simulink library "commfilt2"  (Simulink 6.0)
settings: Solver=ode45  SolverMode=SingleTasking  StartTime=0.0  StopTime=10.0  RelTol=1e-3
undefined symbols (not defined in the file or in its folder): hFilt, rectPul
libraries: dspsigattribs x6, dsparch4 x3, dspsigops x3, dspmlti3 x1
settings Model: Creator=arodrigu  LastModifiedBy=cvora  ExtModeAutoUpdateStatusClock=off  ProdHWDeviceType=Specified
settings DataIOCC: SignalLoggingName=logsOut
settings OptimizationCC: BooleanDataType=off
settings DebuggingCC: CheckExecutionContextPreStartOutputMsg=on  CheckExecutionContextRuntimeOutputMsg=on  SolverPrmCheckMsg=none
settings HardwareCC: ProdHWDeviceType=Specified  TargetUnknown=on
settings ModelReferenceCC: UpdateModelReferenceTargets=IfOutOfDate
settings SFSimCC: SFSimApplyToAllLibs=on  SFSimBuildMode=Incremental

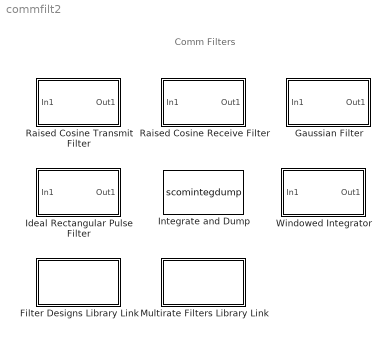
== system commfilt2 ==
  note: Comm Filters
  Filter Designs Library Link : Subsystem  PropExecContextAcrossSSBoundary=on  mask(Link to Filter Designs Library){myFiltDesignsParam=0}
      mask prompts: myFiltDesignsParam "option:"
      settings: OpenFcn=commblkmorefilt('dsparch');
      mask Display: disp('Filter\n Designs Link');
  Gaussian Filter : Subsystem  PropExecContextAcrossSSBoundary=on  mask(Gaussian Filter){N=8, BT=0.3, D=2, sampMode=Frame-based, normMode=Sum of coefficients, filterGain=1, checkCoeff=Off, variableName=gaussFilt, launchFVT=Off}
      mask prompts: N "Input samples per symbol (N):"; BT "BT product:"; D "Group delay (number of symbols):"; sampMode "Input sampling mode:"; normMode "Filter coefficient normalization:"; filterGain "Linear amplitude filter gain:"; checkCoeff "Export filter coefficients to workspace"; variableName "Coefficient variable name:"; launchFVT "Launch Filter Visualization Tool (FVTool)"
      mask help:
      | Filter the input signal using a Gaussian FIR filter.
      |
      | The group delay is specified as the number of symbol periods between the start of the filter response and its peak. This delay also determines the length of the filter impulse response, which is 2 * N * Group delay + 1.
      mask init:
      | [hFilt,icon,msg] = commblkgaussfilt(gcb,'init');
      | if(~isempty(msg))
      | 	error(msg);
      | end
      | 
      | %-- Open FVtool
      | if strcmp(get_param(bdroot(gcb),'simulationstatus'),'stopped')
      | lnkfvtool2mask(gcb);
      | end
      settings: CopyFcn=commblkgaussfilt(gcb,'cbCopyFcn');
      mask Help: helpview(commbhelp);
      mask StyleString: edit,edit,edit,popup(Frame-based|Sample-based),popup(Sum of coefficients|Filter energy|Peak amplitude),edit,checkbox,edit,checkbox
      mask CallbackString: |||commblkgaussfilt(gcb,'cbSampMode');|||commblkgaussfilt(gcb,'cbCheckCoeff');||
      mask Display: plot(0,0,1,1,icon.xx,icon.plot); text(icon.x,icon.y,icon.str,'horiz','center');
  Ideal Rectangular Pulse Filter : Subsystem  PropExecContextAcrossSSBoundary=on  mask(Ideal Rectangular Pulse Filter){pulseLen=8, pulseDelay=0, sampMode=Frame-based, normCheck=on, normMode=Sum of samples, filterGain=1}
      mask prompts: pulseLen "Pulse length (number of samples):"; pulseDelay "Pulse delay (number of samples):"; sampMode "Input sampling mode:"; normCheck "Normalize output signal"; normMode "Normalization method:"; filterGain "Linear amplitude gain:"
      mask help:
      | Upsample the input signal using ideal rectangular pulses.
      |
      | This block replicates each input sample N times, where N is the pulse length. This block can also normalize the output signal and apply a linear amplitude gain.
      mask init:
      | [rectPul,msg] = commblkrectpulse(gcb,'init');
      | if(~isempty(msg))
      | 	error(msg);
      | end
      settings: CopyFcn=commblkrectpulse(gcb,'cbCopyFcn');
      mask Help: helpview(commbhelp);
      mask StyleString: edit,edit,popup(Frame-based|Sample-based),checkbox,popup(Sum of samples|Energy per pulse),edit
      mask CallbackString: ||commblkrectpulse(gcb,'cbSampMode');|commblkrectpulse(gcb,'cbNormCheck');||
      mask Display:
      | plot(0,0,100,100,[95 5 10 10 10 reshape(([85*[0:1/15:1-1/15]+10; 85*[1/15:1/15:1]+10]),1,30)],[75 75 75 70 95 90 90 90 90 90 90 90 90 80 80 80 80 80 80 80 80 80 80 90 90 90 90 90 90 90 90 80 80 80 80]*1.1-10);
      | text(50,35,'Rectangular\nPulse Filter','horiz','center');
  Integrate and Dump : S-Function  FunctionName=scomintegdump  Parameters=obssamples, offsetsamples, nodump  mask(Integrate and dump){obssamples=8, offsetsamples=0, nodump=off}
      mask prompts: obssamples "Integration period (number of samples):"; offsetsamples "Offset (number of samples):"; nodump "Output intermediate values"
      mask help:
      | Integrate over number of samples in integration period and reset at the end of integration.
      |
      | Frame based K x L input is treated as L channels each of frame size K.
      | The samples are integrated along every column.
      |
      | Offset samples are ignored during the first integration period.
      mask Help: helpview(commbhelp);
      mask Display: disp('Integrate\nand Dump')
  Multirate Filters Library Link : Subsystem  PropExecContextAcrossSSBoundary=on  mask(Link to Multirate Filters Library){myMultirateFiltersParam=0}
      mask prompts: myMultirateFiltersParam "option:"
      settings: OpenFcn=commblkmorefilt('dspmlti');
      mask Display: disp('Multirate\nFilters Link');
  Raised Cosine Receive Filter : Subsystem  PropExecContextAcrossSSBoundary=on  mask(Raised Cosine Receive Filter){filtType=Square root, N=8, D=4, R=0.2, sampMode=Frame-based, rateMode=Downsampling, downFactor=8, downOffset=0, checkGain=Normalized, filterGain=1, checkCoeff=off, variableName=rcRxFilt, launchFVT=off}
      mask prompts: filtType "Filter type:"; N "Input samples per symbol (N):"; D "Group delay (number of symbols):"; R "Rolloff factor (0 to 1):"; sampMode "Input sampling mode:"; rateMode "Output mode:"; downFactor "Downsampling factor (L):"; downOffset "Sample offset (0 to L-1):"; checkGain "Filter gain:"; filterGain "Linear amplitude filter gain:"; checkCoeff "Export filter coefficients to workspace"; variableName "Coefficient variable name:"; launchFVT "Launch Filter Visualization Tool (FVTool)"
      mask help:
      | Filter the input signal, and downsample if selected, using a normal or square root raised cosine FIR filter.
      |
      | The group delay is specified as the number of symbol periods between the start of the filter response and its peak. This delay also determines the length of the filter impulse response, which is 2 * N * Group delay + 1.
      |
      | In normalized mode, the coefficients of the normal raised cosine filter are normalized so that the peak coefficient is equal to one. The filter coefficients of the square root raised cosine filter are normalized so that the impulse response of the filter convolved with itself is approximately the impulse response of the normal filter.
      mask init:
      | [hFilt,icon,msg] = commblkrcfilt(gcb,'init','RX');
      | if(~isempty(msg))
      | 	error(msg);
      | end
      | 
      | %-- Open FVtool
      | if strcmp(get_param(bdroot(gcb),'simulationstatus'),'stopped')
      | lnkfvtool2mask(gcb);
      | end
      settings: CopyFcn=commblkrcfilt(gcb,'cbCopyFcn');
      mask Help: helpview(commbhelp);
      mask StyleString: popup(Normal|Square root),edit,edit,edit,popup(Frame-based|Sample-based),popup(Downsampling|None),edit,edit,popup(Normalized|User-specified),edit,checkbox,edit,checkbox
      mask CallbackString: ||||commblkrcfilt(gcb,'cbSampMode','RX');|commblkrcfilt(gcb,'cbRateMode');|||commblkrcfilt(gcb,'cbCheckGain');||commblkrcfilt(gcb,'cbCheckCoeff');||
      mask Display: plot(0,0,1,1,icon.xx,icon.plot); text(icon.x,icon.y,icon.str,'horiz','center');
  Raised Cosine Transmit Filter : Subsystem  PropExecContextAcrossSSBoundary=on  mask(Raised Cosine Transmit Filter){filtType=Square root, D=4, R=0.2, sampMode=Frame-based, N=8, checkGain=Normalized, filterGain=1, checkCoeff=off, variableName=rcTxFilt, launchFVT=off}
      mask prompts: filtType "Filter type:"; D "Group delay (number of symbols):"; R "Rolloff factor (0 to 1):"; sampMode "Input sampling mode:"; N "Upsampling factor (N):"; checkGain "Filter gain:"; filterGain "Linear amplitude filter gain:"; checkCoeff "Export filter coefficients to workspace"; variableName "Coefficient variable name:"; launchFVT "Launch Filter Visualization Tool (FVTool)"
      mask help:
      | Upsample and filter the input signal using a normal or square root raised cosine FIR filter.
      |
      | The group delay is specified as the number of symbol periods between the start of the filter response and its peak. This delay also determines the length of the filter impulse response, which is 2 * N * Group delay + 1.
      |
      | In normalized mode, the coefficients of the normal raised cosine filter are normalized so that the peak coefficient is equal to one. The filter coefficients of the square root raised cosine filter are normalized so that the impulse response of the filter convolved with itself is approximately the impulse response of the normal filter.
      mask init:
      | [hFilt,icon,msg] = commblkrcfilt(gcb,'init','TX');
      | if(~isempty(msg))
      | 	error(msg);
      | end
      | 
      | %-- Open FVtool
      | if strcmp(get_param(bdroot(gcb),'simulationstatus'),'stopped')
      | lnkfvtool2mask(gcb);
      | end
      settings: CopyFcn=commblkrcfilt(gcb,'cbCopyFcn');
      mask Help: helpview(commbhelp);
      mask StyleString: popup(Normal|Square root),edit,edit,popup(Frame-based|Sample-based),edit,popup(Normalized|User-specified),edit,checkbox,edit,checkbox
      mask CallbackString: |||commblkrcfilt(gcb,'cbSampMode','TX');||commblkrcfilt(gcb,'cbCheckGain');||commblkrcfilt(gcb,'cbCheckCoeff');||
      mask Display: plot(0,0,1,1,icon.xx,icon.plot); text(icon.x,icon.y,icon.str,'horiz','center');
  Windowed Integrator : Subsystem  PropExecContextAcrossSSBoundary=on  mask(Windowed Integrator){integperiod=8}
      mask prompts: integperiod "Integration period (number of samples):"
      mask help: Integrate a discrete input signal over the sliding window of size equal to the integration period.
      mask init:
      | msg = commblkwininteg(gcb);
      | if(~isempty(msg))
      | 	error(msg);
      | end
      settings: ErrorFcn=commblkwinintegchk
      mask Help: helpview(commbhelp);
      mask Display: disp('Windowed\nIntegrator');

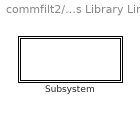
== system commfilt2/Filter Designs Library Link ==
  Subsystem : Subsystem  PropExecContextAcrossSSBoundary=on
      mask Display: disp(' ')

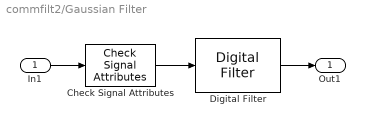
== system commfilt2/Gaussian Filter ==
  In1 : Inport  LatchInput=off
  Check Signal Attributes : dspsigattribs/Check Signal Attributes  SigAttribCheckMethod=Does not match attributes exactly  Complexity=Ignore  Frame=Frame-based  DimsCheckMethod=Is...  Dimensions=Column vector (2-D) or scalar  DatatypeCheckMethod=Ignore  DatatypeGeneral=Boolean  DtypeFloatSpecific=Any floating-point  DtypeFixedSpecific=Any fixed-point  DtypeIntSpecific=Any integer  SampleMode=Ignore
  Digital Filter : dsparch4/Digital Filter  TypePopup=FIR (all zeros)  IIRFiltStruct=Direct form II transposed  AllPoleFiltStruct=Direct form  FIRFiltStruct=Direct form  CoeffSource=Specify via dialog  NumCoeffs=hFilt.coeff  DenCoeffs=[1]  BiQuadCoeffs=[1 0.3 0.4 1 0.1 0.2]  LatticeCoeffs=[0.2 0.4]  denIgnore=on  FiltPerSampPopup=One filter per frame  IC=0  ICnum=0  ICden=0  roundingMode=Floor  overflowMode=off
  Out1 : Outport
  wires:
  Digital Filter/1 -> Out1/1
  Check Signal Attributes/1 -> Digital Filter/1
  In1/1 -> Check Signal Attributes/1

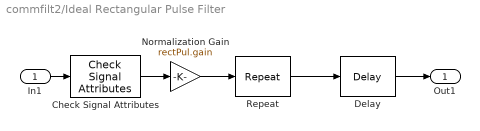
== system commfilt2/Ideal Rectangular Pulse Filter ==
  In1 : Inport  LatchInput=off
  Check Signal Attributes : dspsigattribs/Check Signal Attributes  SigAttribCheckMethod=Does not match attributes exactly  Complexity=Ignore  Frame=Frame-based  DimsCheckMethod=Is...  Dimensions=Column vector (2-D) or scalar  DatatypeCheckMethod=Ignore  DatatypeGeneral=Boolean  DtypeFloatSpecific=Any floating-point  DtypeFixedSpecific=Any fixed-point  DtypeIntSpecific=Any integer  SampleMode=Ignore
  Delay : dspsigops/Delay  dly_unit=Samples  delay=rectPul.pulseDelay  ic_detail=off  dif_ic_for_ch=off  dif_ic_for_dly=off  ic=0  reset_popup=None
  Normalization Gain : Gain  Gain=rectPul.gain  SaturateOnIntegerOverflow=on
  Repeat : dspsigops/Repeat  N=rectPul.pulseLen  ic=0  mode=Maintain input frame rate
  Out1 : Outport
  wires:
  Delay/1 -> Out1/1
  Normalization Gain/1 -> Repeat/1
  In1/1 -> Check Signal Attributes/1
  Repeat/1 -> Delay/1
  Check Signal Attributes/1 -> Normalization Gain/1

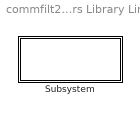
== system commfilt2/Multirate Filters Library Link ==
  Subsystem : Subsystem  PropExecContextAcrossSSBoundary=on
      mask Display: disp(' ')

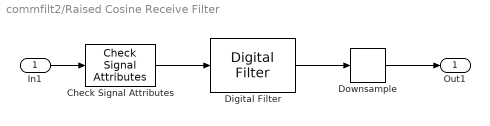
== system commfilt2/Raised Cosine Receive Filter ==
  In1 : Inport  LatchInput=off
  Check Signal Attributes : dspsigattribs/Check Signal Attributes  SigAttribCheckMethod=Does not match attributes exactly  Complexity=Ignore  Frame=Frame-based  DimsCheckMethod=Is...  Dimensions=Column vector (2-D) or scalar  DatatypeCheckMethod=Ignore  DatatypeGeneral=Boolean  DtypeFloatSpecific=Any floating-point  DtypeFixedSpecific=Any fixed-point  DtypeIntSpecific=Any integer  SampleMode=Ignore
  Digital Filter : dsparch4/Digital Filter  TypePopup=FIR (all zeros)  IIRFiltStruct=Direct form II transposed  AllPoleFiltStruct=Direct form  FIRFiltStruct=Direct form  CoeffSource=Specify via dialog  NumCoeffs=hFilt.coeff  DenCoeffs=[1]  BiQuadCoeffs=[1 0.3 0.4 1 0.1 0.2]  LatticeCoeffs=[0.2 0.4]  denIgnore=on  FiltPerSampPopup=One filter per frame  IC=0  ICnum=0  ICden=0  roundingMode=Floor  overflowMode=off
  Downsample : dspsigops/Downsample  N=hFilt.rateFactor  phase=hFilt.downOffset  ic=0  smode=Allow multirate  fmode=Maintain input frame rate
  Out1 : Outport
  wires:
  Digital Filter/1 -> Downsample/1
  Downsample/1 -> Out1/1
  Check Signal Attributes/1 -> Digital Filter/1
  In1/1 -> Check Signal Attributes/1

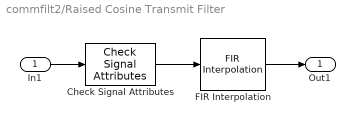
== system commfilt2/Raised Cosine Transmit Filter ==
  In1 : Inport  LatchInput=off
  Check Signal Attributes : dspsigattribs/Check Signal Attributes  SigAttribCheckMethod=Does not match attributes exactly  Complexity=Ignore  Frame=Frame-based  DimsCheckMethod=Is...  Dimensions=Column vector (2-D) or scalar  DatatypeCheckMethod=Ignore  DatatypeGeneral=Boolean  DtypeFloatSpecific=Any floating-point  DtypeFixedSpecific=Any fixed-point  DtypeIntSpecific=Any integer  SampleMode=Ignore
  FIR Interpolation : dspmlti3/FIR Interpolation  DialogController=dspDDGCreate  DialogControllerArgs=DataTag0  h=hFilt.coeff  L=hFilt.rateFactor  framing=Maintain input frame rate  outputBufInitCond=0  roundingMode=Floor  overflowMode=off
  Out1 : Outport
  wires:
  In1/1 -> Check Signal Attributes/1
  Check Signal Attributes/1 -> FIR Interpolation/1
  FIR Interpolation/1 -> Out1/1

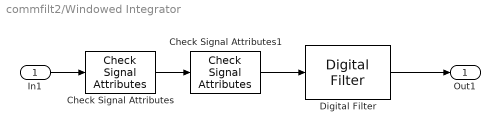
== system commfilt2/Windowed Integrator ==
  In1 : Inport  LatchInput=off
  Check Signal Attributes : dspsigattribs/Check Signal Attributes  SigAttribCheckMethod=Matches attributes exactly  Complexity=Ignore  Frame=Sample-based  DimsCheckMethod=Is...  Dimensions=Vector (1-D or 2-D)  DatatypeCheckMethod=Ignore  DatatypeGeneral=Boolean  DtypeFloatSpecific=Any floating-point  DtypeFixedSpecific=Any fixed-point  DtypeIntSpecific=Any integer  SampleMode=Ignore
  Check Signal Attributes1 : dspsigattribs/Check Signal Attributes  SigAttribCheckMethod=Matches attributes exactly  Complexity=Ignore  Frame=Sample-based  DimsCheckMethod=Is...  Dimensions=Full matrix (2-D)  DatatypeCheckMethod=Ignore  DatatypeGeneral=Boolean  DtypeFloatSpecific=Any floating-point  DtypeFixedSpecific=Any fixed-point  DtypeIntSpecific=Any integer  SampleMode=Ignore
  Digital Filter : dsparch4/Digital Filter  DialogController=dspDDGCreate  DialogControllerArgs=DataTag1  TypePopup=FIR (all zeros)  IIRFiltStruct=Direct form I  AllPoleFiltStruct=Direct form  FIRFiltStruct=Direct form  CoeffSource=Specify via dialog  NumCoeffs=ones(1,integperiod)  DenCoeffs=1  BiQuadCoeffs=[1 0.3 0.4 1 0.1 0.2]  LatticeCoeffs=[0.2 0.4]  denIgnore=on  FiltPerSampPopup=One filter per frame  IC=0  ICnum=0  ICden=0  roundingMode=Floor  overflowMode=off  ScaleValues=1  scaleValueFracLength=14  stageInFracLength=15  stageOutFracLength=15
  Out1 : Outport
  wires:
  Check Signal Attributes/1 -> Check Signal Attributes1/1
  Digital Filter/1 -> Out1/1
  In1/1 -> Check Signal Attributes/1
  Check Signal Attributes1/1 -> Digital Filter/1

== system commfilt2/Filter Designs Library Link/Subsystem ==

== system commfilt2/Multirate Filters Library Link/Subsystem ==
